simulink model "impedance_control"  (R2023b)
settings: Solver=VariableStepAuto  StartTime=0.0  StopTime=2  RelTol=1e-3
values from neighbouring files (symbols this model uses):
  Tc = 0.0005    [state.m]
settings Model: Creator=blankyw  LastModifiedBy=blankyw

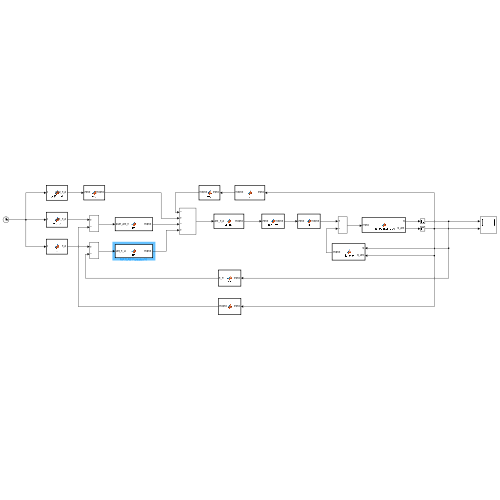
[thumbnail: Simulink's stored preview of the top-level diagram]
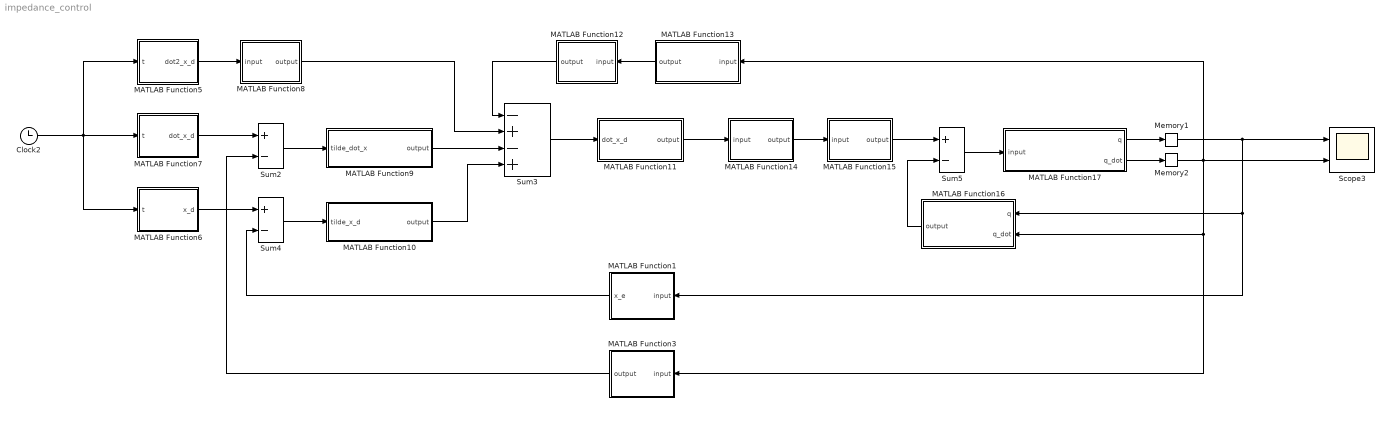
== system impedance_control ==
  Clock2 : Clock
  MATLAB Function1 : MATLAB Function  TreatAsAtomicUnit=on
  MATLAB Function10 : MATLAB Function  TreatAsAtomicUnit=on
  MATLAB Function11 : MATLAB Function  TreatAsAtomicUnit=on
  MATLAB Function12 : MATLAB Function  TreatAsAtomicUnit=on
  MATLAB Function13 : MATLAB Function  TreatAsAtomicUnit=on
  MATLAB Function14 : MATLAB Function  TreatAsAtomicUnit=on
  MATLAB Function15 : MATLAB Function  TreatAsAtomicUnit=on
  MATLAB Function16 : MATLAB Function  TreatAsAtomicUnit=on
  MATLAB Function17 : MATLAB Function  TreatAsAtomicUnit=on
  MATLAB Function3 : MATLAB Function  TreatAsAtomicUnit=on
  MATLAB Function5 : MATLAB Function  TreatAsAtomicUnit=on
  MATLAB Function6 : MATLAB Function  TreatAsAtomicUnit=on
  MATLAB Function7 : MATLAB Function  TreatAsAtomicUnit=on
  MATLAB Function8 : MATLAB Function  TreatAsAtomicUnit=on
  MATLAB Function9 : MATLAB Function  TreatAsAtomicUnit=on
  Memory1 : Memory
  Memory2 : Memory
  Scope3 : Scope  NumInputPorts=2
  Sum2 : Sum  Inputs=+-  InputSameDT=on  SaturateOnIntegerOverflow=on  SampleTime=Tc  OutDataTypeStr=Inherit: Same as first input
  Sum3 : Sum  Inputs=-+-+  InputSameDT=on  SaturateOnIntegerOverflow=on  SampleTime=Tc  OutDataTypeStr=Inherit: Same as first input
  Sum4 : Sum  Inputs=+-  InputSameDT=on  SaturateOnIntegerOverflow=on  SampleTime=Tc  OutDataTypeStr=Inherit: Same as first input
  Sum5 : Sum  Inputs=+-  InputSameDT=on  SaturateOnIntegerOverflow=on  SampleTime=Tc  OutDataTypeStr=Inherit: Same as first input
  wires:
  Clock2/1 -> MATLAB Function6/1(t), MATLAB Function5/1(t), MATLAB Function7/1(t)
  MATLAB Function5/1(dot2_x_d) -> MATLAB Function8/1(input)
  MATLAB Function7/1(dot_x_d) -> Sum2/1
  MATLAB Function6/1(x_d) -> Sum4/1
  Sum2/1 -> MATLAB Function9/1(tilde_dot_x)
  Sum4/1 -> MATLAB Function10/1(tilde_x_d)
  MATLAB Function8/1(output) -> Sum3/2
  MATLAB Function9/1(output) -> Sum3/3
  MATLAB Function10/1(output) -> Sum3/4
  Sum3/1 -> MATLAB Function11/1(dot_x_d)
  MATLAB Function12/1(output) -> Sum3/1
  MATLAB Function13/1(output) -> MATLAB Function12/1(input)
  MATLAB Function11/1(output) -> MATLAB Function14/1(input)
  MATLAB Function14/1(output) -> MATLAB Function15/1(input)
  MATLAB Function15/1(output) -> Sum5/1
  MATLAB Function16/1(output) -> Sum5/2
  Sum5/1 -> MATLAB Function17/1(input)
  MATLAB Function1/1(x_e) -> Sum4/2
  MATLAB Function3/1(output) -> Sum2/2
  MATLAB Function17/1(q) -> Memory1/1
  MATLAB Function17/2(q_dot) -> Memory2/1
  Memory2/1 -> MATLAB Function3/1(input), MATLAB Function16/2(q_dot), Scope3/2, MATLAB Function13/1(input)
  Memory1/1 -> MATLAB Function1/1(input), MATLAB Function16/1(q), Scope3/1

== matlab function impedance_control/MATLAB Function16 ==
  data: output output; q input; q_dot input
function output = n_function(q, q_dot)
    n_mat = n;

    output = n_mat;
end

== matlab function impedance_control/MATLAB Function17 ==
  data: q output; input input; q_dot output
function [q, q_dot]= manipulator_dyn(input)
    B_mat = B;

    output = B_mat * input;
end

== matlab function impedance_control/MATLAB Function1 ==
  data: x_e output; input input
function x_e = FK(input)

    x_e = input;
end

== matlab function impedance_control/MATLAB Function3 ==
  data: output output; input input
function output = J(input)

end

== matlab function impedance_control/MATLAB Function5 ==
  data: dot2_x_d output; t input
function dot2_x_d = dot2_x_d(t)

    dot2_x_d = [0; 0; 0];
end

== matlab function impedance_control/MATLAB Function6 ==
  data: x_d output; t input
function x_d = x_d(t)

    x_d = [1; 1; 1];
end

== matlab function impedance_control/MATLAB Function7 ==
  data: dot_x_d output; t input
function dot_x_d = dot_x_d(t)

    dot_x_d = [0; 0; 0];
end

== matlab function impedance_control/MATLAB Function8 ==
  data: output output; input input
function output = md(input)
    md_mat = md;

    output = md_mat * input;
end

== matlab function impedance_control/MATLAB Function9 ==
  data: output output; tilde_dot_x input
function output = kd(tilde_dot_x)
    kd = [1, 0, 0;0, 1, 0;0, 0, 1];

    output = kd * tilde_dot_x;
end

== matlab function impedance_control/MATLAB Function10 ==
  data: output output; tilde_x_d input
function output = kp(tilde_x_d)
    kp = [1, 0, 0;0, 1, 0;0, 0, 1];

    output = kp * tilde_x_d;
end

== matlab function impedance_control/MATLAB Function11 ==
  data: output output; dot_x_d input
function output = J_inv(dot_x_d)

    output = kd * dot_x_d;
end

== matlab function impedance_control/MATLAB Function12 ==
  data: output output; input input
function output = md(input)
    md_mat = md;

    output = md_mat * input;
end

== matlab function impedance_control/MATLAB Function13 ==
  data: output output; input input
function output = J(input)

end

== matlab function impedance_control/MATLAB Function14 ==
  data: output output; input input
function output = md_inv(input)
    md_inv_mat = md_inv;

    output = md_inv_mat * input;
end

== matlab function impedance_control/MATLAB Function15 ==
  data: output output; input input
function output = B(input)
    B_mat = B;

    output = B_mat * input;
end
